simulink model "untitled"  (R2023b)
settings: Solver=VariableStepAuto  StartTime=0.0  StopTime=10  RelTol=1e-3
undefined symbols (not defined in the file): A, c, f, Lp, Ls, Ts
settings Model: Creator=nurbi  LastModifiedBy=nurbi

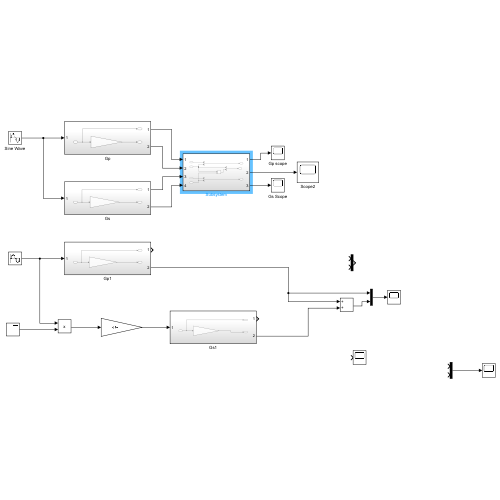
[thumbnail: Simulink's stored preview of the top-level diagram]
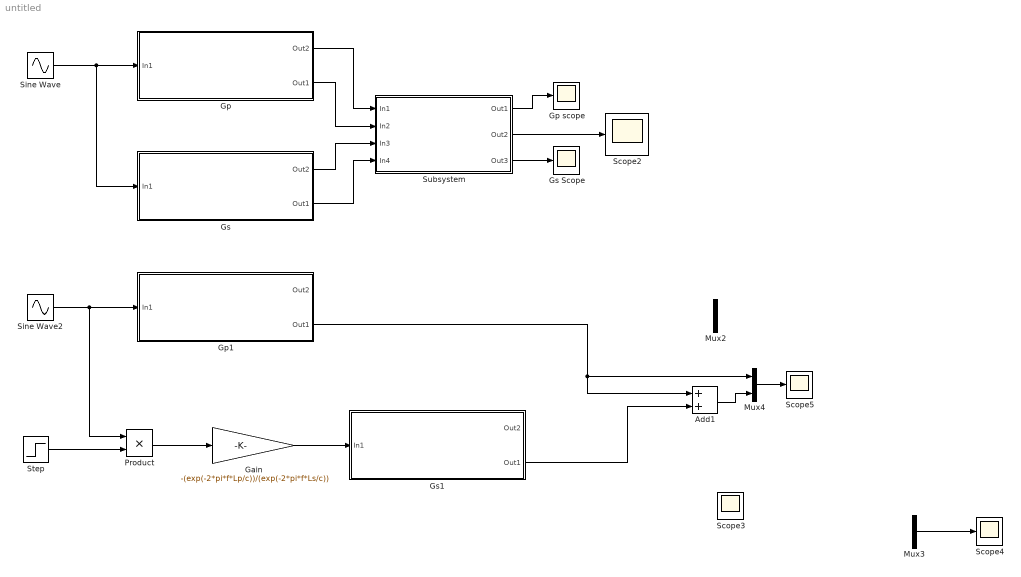
== system untitled ==
  Add1 : Sum
  Gain : Gain  Gain=-(exp(-2*pi*f*Lp/c))/(exp(-2*pi*f*Ls/c))
  Gp : Subsystem
  Gp scope : Scope
  Gp1 : Subsystem
  Gs : Subsystem
  Gs Scope : Scope
  Gs1 : Subsystem
  Mux2 : Mux  Inputs=2
  Mux3 : Mux  Inputs=2
  Mux4 : Mux  Inputs=2
  Product : Product
  Scope{2..5} (4 alike) : Scope
  Sine Wave : Sin  Amplitude=A  Frequency=2*pi*f  SampleTime=Ts
  Sine Wave2 : Sin  Amplitude=A  Frequency=2*pi*f  SampleTime=Ts
  Step : Step  Time=step  SampleTime=0
  Subsystem : Subsystem
  wires:
  Mux3/1 -> Scope4/1
  Sine Wave2/1 -> Gp1/1(In1), Product/1
  Gain/1 -> Gs1/1(In1)
  Mux4/1 -> Scope5/1
  Add1/1 -> Mux4/2
  Step/1 -> Product/2
  Product/1 -> Gain/1
  Sine Wave/1 -> Gs/1(In1), Gp/1(In1)
  Gp/1(Out2) -> Subsystem/1(In1)
  Gp/2(Out1) -> Subsystem/2(In2)
  Gs/1(Out2) -> Subsystem/3(In3)
  Gs/2(Out1) -> Subsystem/4(In4)
  Subsystem/1(Out1) -> Gp scope/1
  Subsystem/2(Out2) -> Scope2/1
  Subsystem/3(Out3) -> Gs Scope/1
  Gs1/2(Out1) -> Add1/2
  Gp1/2(Out1) -> Mux4/1, Add1/1

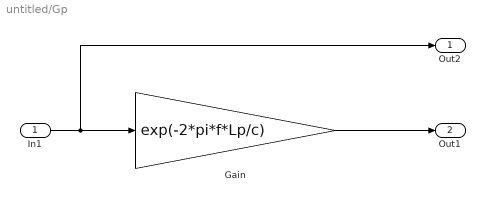
== system untitled/Gp ==
  In1 : Inport
  Gain : Gain  Gain=exp(-2*pi*f*Lp/c)
  Out2 : Outport
  Out1 : Outport  Port=2
  wires:
  In1/1 -> Out2/1, Gain/1
  Gain/1 -> Out1/1

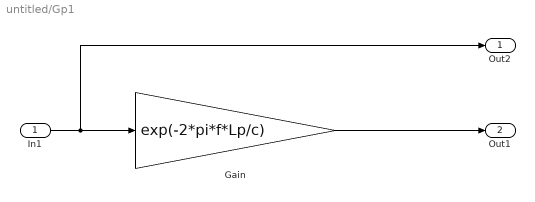
== system untitled/Gp1 ==
  In1 : Inport
  Gain : Gain  Gain=exp(-2*pi*f*Lp/c)
  Out2 : Outport
  Out1 : Outport  Port=2
  wires:
  In1/1 -> Out2/1, Gain/1
  Gain/1 -> Out1/1

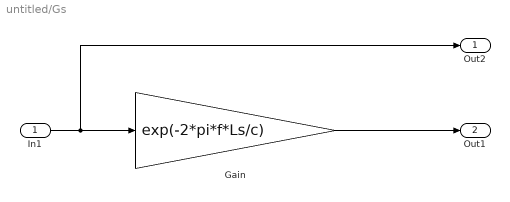
== system untitled/Gs ==
  In1 : Inport
  Gain : Gain  Gain=exp(-2*pi*f*Ls/c)
  Out2 : Outport
  Out1 : Outport  Port=2
  wires:
  In1/1 -> Out2/1, Gain/1
  Gain/1 -> Out1/1

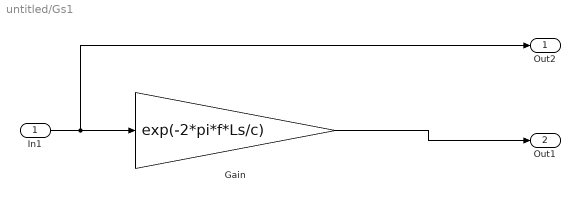
== system untitled/Gs1 ==
  In1 : Inport
  Gain : Gain  Gain=exp(-2*pi*f*Ls/c)
  Out2 : Outport
  Out1 : Outport  Port=2
  wires:
  In1/1 -> Out2/1, Gain/1
  Gain/1 -> Out1/1

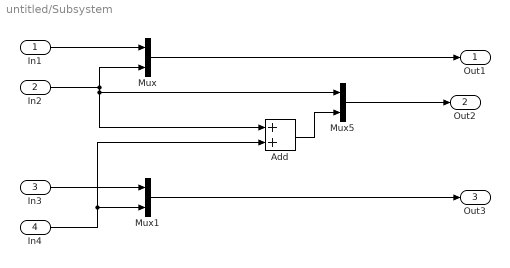
== system untitled/Subsystem ==
  In1 : Inport
  In2 : Inport  Port=2
  In3 : Inport  Port=3
  In4 : Inport  Port=4
  Add : Sum
  Mux : Mux  Inputs=2
  Mux1 : Mux  Inputs=2
  Mux5 : Mux  Inputs=2
  Out1 : Outport
  Out2 : Outport  Port=2
  Out3 : Outport  Port=3
  wires:
  Mux/1 -> Out1/1
  Mux5/1 -> Out2/1
  In3/1 -> Mux1/1
  Mux1/1 -> Out3/1
  In2/1 -> Add/1, Mux5/1, Mux/2
  In4/1 -> Mux1/2, Add/2
  In1/1 -> Mux/1
  Add/1 -> Mux5/2
